simulink model "LoadControl"  (R2013a)
settings: Solver=ode45  StartTime=0.0  StopTime=0.2  RelTol=1e-3
settings Model: CovMetricSettings=drw  CovHTMLOptions=-sRT=1 -aTS=1 -bRG=1 -bTC=1 -hTR=0 -nFC=0 -scm=1 -bcm=1 -xEv=0  CovExternalEMLEnable=on  Creator=MEHEDI HASSAN  LastModifiedBy=Mohiuddin Muztaba
settings DebuggingCC: SolverPrmCheckMsg=none  ModelReferenceExtraNoncontSigs=none

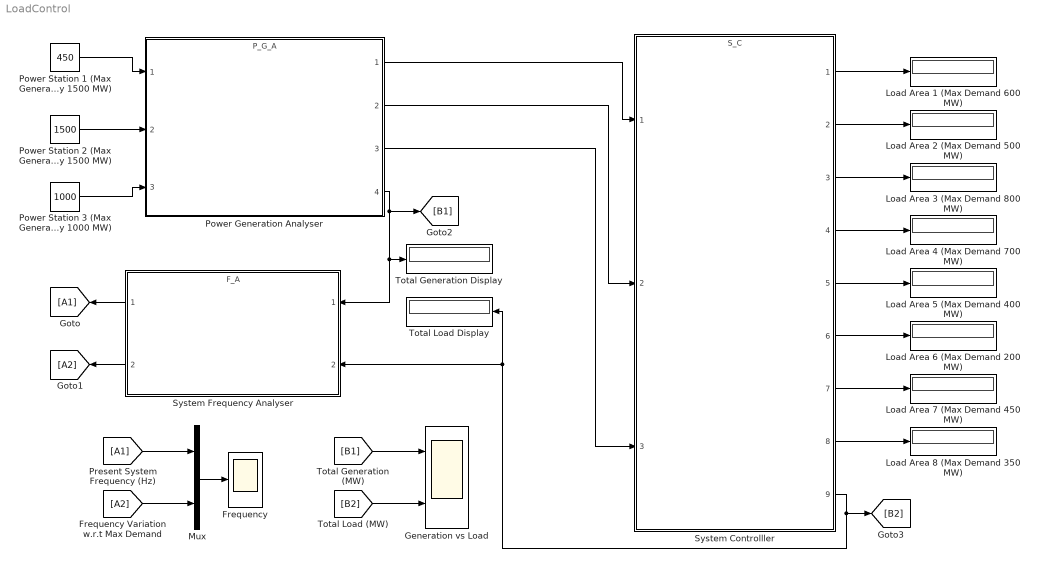
== system LoadControl ==
  Frequency : Scope
      settings: TickLabels=on  ShowLegends=on
  Generation vs Load : Scope  NumInputPorts=2
      settings: ShowLegends=on  YMin=-5~-5  YMax=5~5
  Load Area 1 (Max Demand 600 MW) : Display
  Load Area 2 (Max Demand 500 MW) : Display
  Load Area 3 (Max Demand 800 MW) : Display
  Load Area 4 (Max Demand 700 MW) : Display
  Load Area 5 (Max Demand 400 MW) : Display
  Load Area 6 (Max Demand 200 MW) : Display
  Load Area 7 (Max Demand 450 MW) : Display
  Load Area 8 (Max Demand 350 MW) : Display
  Mux : Mux  Inputs=2
  Power Generation Analyser : ModelReference  ModelNameDialog=P_G_A.slx  SimulationMode=Normal  ModelReferenceVersion=1.15  CopyOfModelName=P_G_A.slx  DefaultDataLogging=on
  Power Station 1 (Max Generation Capacity 1500 MW) : Constant  Value=450
  Power Station 2 (Max Generation Capacity 1500 MW) : Constant  Value=1500
  Power Station 3 (Max Generation Capacity 1000 MW) : Constant  Value=1000
  System Controlller : ModelReference  ModelNameDialog=S_C.slx  SimulationMode=Normal  ModelReferenceVersion=1.12  CopyOfModelName=S_C.slx  DefaultDataLogging=on
  System Frequency Analyser : ModelReference  ModelNameDialog=F_A.slx  SimulationMode=Normal  ModelReferenceVersion=1.5  CopyOfModelName=F_A.slx  DefaultDataLogging=on
  Total Generation Display : Display
  Total Load Display : Display
  wires:
  Power Station 1 (Max Generation Capacity 1500 MW)/1 -> Power Generation Analyser/1
  Power Station 2 (Max Generation Capacity 1500 MW)/1 -> Power Generation Analyser/2
  Power Station 3 (Max Generation Capacity 1000 MW)/1 -> Power Generation Analyser/3
  Power Generation Analyser/1 -> System Controlller/1
  Power Generation Analyser/2 -> System Controlller/2
  Power Generation Analyser/3 -> System Controlller/3
  Mux/1 -> Frequency/1
  Power Generation Analyser/4 -> Total Generation Display/1, System Frequency Analyser/1, [B1]
  System Controlller/9 -> [B2], Total Load Display/1, System Frequency Analyser/2
  System Controlller/1 -> Load Area 1 (Max Demand 600 MW)/1
  System Controlller/2 -> Load Area 2 (Max Demand 500 MW)/1
  System Controlller/3 -> Load Area 3 (Max Demand 800 MW)/1
  System Controlller/4 -> Load Area 4 (Max Demand 700 MW)/1
  System Controlller/5 -> Load Area 5 (Max Demand 400 MW)/1
  System Controlller/6 -> Load Area 6 (Max Demand 200 MW)/1
  System Controlller/7 -> Load Area 7 (Max Demand 450 MW)/1
  System Controlller/8 -> Load Area 8 (Max Demand 350 MW)/1
  System Frequency Analyser/1 -> [A1]
  System Frequency Analyser/2 -> [A2]
  [B1] -> Generation vs Load/1
  [B2] -> Generation vs Load/2
  [A1] -> Mux/1
  [A2] -> Mux/2
